simulink model "eval_ekf"  (R2026a)
settings: Solver=VariableStepAuto  StopTime=1000
undefined symbols (not defined in the file): ekf_param, pf_param, plant_param, r_param
libraries: lib_sensors x3, lib_plant x1
settings Model: SimulationMode=accelerator  Creator=alessandro-nardin  LastModifiedBy=alessandro-nardin
settings RTWCC: Toolchain=Microsoft Visual C++ 2022 v17.0 | nmake (64-bit Windows)

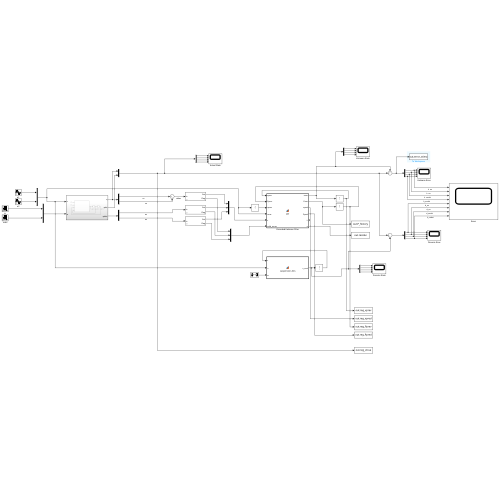
[thumbnail: Simulink's stored preview of the top-level diagram]
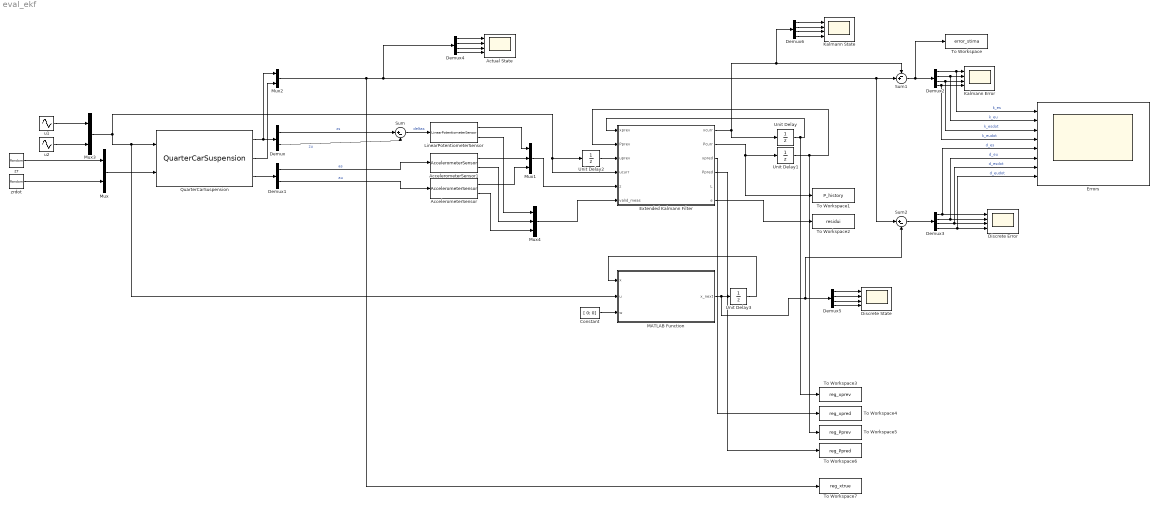
== system eval_ekf ==
  AccelerometerSensor : lib_sensors/AccelerometerSensor  out_sample_t=1/ekf_param.freq
  AccelerometerSensor1 : lib_sensors/AccelerometerSensor  out_sample_t=1/ekf_param.freq
  Actual State : Scope  NumInputPorts=4
      settings: ActiveDisplayYMinimum=-13.406936930450598  ActiveDisplayYMaximum=16.431517639223237  DataLoggingVariableName=ScopeData2
  Constant : Constant  Value=[ 0; 0]
  Demux : Demux  Outputs=2
  Demux1 : Demux  Outputs=2
  Demux{2..6} (5 alike) : Demux
  Discrete Error : Scope  NumInputPorts=4
      settings: ActiveDisplayYMinimum=-0.13461336894615539  ActiveDisplayYMaximum=0.12972172873522425
  Discrete State : Scope  NumInputPorts=4
      settings: ActiveDisplayYMinimum=-16.662431963356159  ActiveDisplayYMaximum=16.863664846001409  DataLoggingVariableName=ScopeData3
  Errors : Scope  NumInputPorts=8
      settings: ActiveDisplayYMinimum=-0.11152200034289453  ActiveDisplayYMaximum=0.13726275911567587  DataLoggingVariableName=ScopeData5
  Extended Kalmann Filter : MATLAB Function  TreatAsAtomicUnit=on
  Kalmann Error : Scope  NumInputPorts=4
      settings: ActiveDisplayYMinimum=-0.727367767410682  ActiveDisplayYMaximum=0.68734917974136311
  Kalmann State : Scope  NumInputPorts=4
      settings: ActiveDisplayYMinimum=-12.347879763067127  ActiveDisplayYMaximum=15.301795380492928  DataLoggingVariableName=ScopeData4
  LinearPotentiometerSensor : lib_sensors/LinearPotentiometerSensor  out_sample_t=1/ekf_param.freq
  MATLAB Function : MATLAB Function  TreatAsAtomicUnit=on
  Mux : Mux  Inputs=2
  Mux1 : Mux  Inputs=3
  Mux2 : Mux  Inputs=2
  Mux3 : Mux  Inputs=2
  Mux4 : Mux  Inputs=3
  QuarterCarSuspension : lib_plant/QuarterCarSuspension  SystemSampleTime=-1  VariantActivationTime=update diagram  EmptyChoice=off  PassThrough=off  PassThroughVariantControl=(default)  EmptyChoiceVariantControl=(default)  AllowFlexibleInterface=on  Latency=0  AutoFrameSizeCalculation=off
      settings: SourceProductName=Lib Plant
  Sum : Sum  Inputs=|+-
  Sum1 : Sum  Inputs=-+|
  Sum2 : Sum  Inputs=|+-
  To Workspace : ToWorkspace  VariableName=error_stima  SaveFormat=Timeseries  SampleTime=pf_param.sample_t
  To Workspace1 : ToWorkspace  VariableName=P_history  SaveFormat=Timeseries  SampleTime=-1
  To Workspace2 : ToWorkspace  VariableName=residui  SaveFormat=Timeseries  SampleTime=-1
  To Workspace3 : ToWorkspace  VariableName=reg_xprev  SaveFormat=Timeseries  SampleTime=1/ekf_param.freq
  To Workspace4 : ToWorkspace  VariableName=reg_xpred  SaveFormat=Timeseries  SampleTime=1/ekf_param.freq
  To Workspace5 : ToWorkspace  VariableName=reg_Pprev  SaveFormat=Timeseries  SampleTime=1/ekf_param.freq
  To Workspace6 : ToWorkspace  VariableName=reg_Ppred  SaveFormat=Timeseries  SampleTime=1/ekf_param.freq
  To Workspace7 : ToWorkspace  VariableName=reg_xtrue  SaveFormat=Timeseries  SampleTime=1/ekf_param.freq
  Unit Delay : UnitDelay  InitialCondition=ekf_param.x_init  SampleTime=ekf_param.sample_t
  Unit Delay1 : UnitDelay  InitialCondition=ekf_param.P_init  SampleTime=ekf_param.sample_t
  Unit Delay2 : UnitDelay  InitialCondition=[ 0; 0]  SampleTime=ekf_param.sample_t
  Unit Delay3 : UnitDelay  InitialCondition=ekf_param.x_init  SampleTime=-1
  u1 : Sin  Amplitude=943  Frequency=0.5  Phase=0.2  SampleTime=0
  u2 : Sin  Amplitude=2000  Phase=1  SampleTime=0
  zr : RandomNumber  Variance=r_param.rz_var  Seed=3245  SampleTime=0
  zrdot : RandomNumber  Variance=r_param.rzdot_var  Seed=213  SampleTime=0
  wires:
  QuarterCarSuspension/1 -> Demux/1, Mux2/1
  Demux/1 -> Sum/1  "zs"
  Demux/2 -> Sum/2  "zu"
  Sum/1 -> LinearPotentiometerSensor/1  "deltas"
  Demux1/2 -> AccelerometerSensor/1  "au"
  QuarterCarSuspension/3 -> Demux1/1
  Demux1/1 -> AccelerometerSensor1/1  "as"
  Mux/1 -> QuarterCarSuspension/2
  Extended Kalmann Filter/2(Pcurr) -> To Workspace1/1, Unit Delay1/1
  Unit Delay1/1 -> To Workspace5/1, Extended Kalmann Filter/2(Pprev)
  Mux3/1 -> QuarterCarSuspension/1, MATLAB Function/2(u), Extended Kalmann Filter/4(ucurr), Unit Delay2/1
  Unit Delay2/1 -> Extended Kalmann Filter/3(uprev)
  AccelerometerSensor1/1 -> Mux1/2
  Mux1/1 -> Extended Kalmann Filter/5(z)
  zr/1 -> Mux/1
  zrdot/1 -> Mux/2
  Unit Delay/1 -> To Workspace3/1, Extended Kalmann Filter/1(xprev)
  u1/1 -> Mux3/1
  u2/1 -> Mux3/2
  Unit Delay3/1 -> MATLAB Function/1(x)
  Constant/1 -> MATLAB Function/3(w)
  QuarterCarSuspension/2 -> Mux2/2
  Sum1/1 -> To Workspace/1, Demux2/1
  Demux2/1 -> Errors/1, Kalmann Error/1  "k_es"
  Demux2/2 -> Errors/2, Kalmann Error/2  "k_eu"
  Demux2/3 -> Errors/3, Kalmann Error/3  "k_esdot"
  Demux2/4 -> Errors/4, Kalmann Error/4  "k_eudot"
  Sum2/1 -> Demux3/1
  Demux3/4 -> Errors/8, Discrete Error/4  "d_eudot"
  Demux3/2 -> Errors/6, Discrete Error/2  "d_eu"
  Demux3/1 -> Errors/5, Discrete Error/1  "d_es"
  Demux3/3 -> Errors/7, Discrete Error/3  "d_esdot"
  Demux4/4 -> Actual State/4
  Mux2/1 -> To Workspace7/1, Demux4/1, Sum1/2, Sum2/1
  Demux4/2 -> Actual State/2
  Demux4/3 -> Actual State/3
  Demux4/1 -> Actual State/1
  Demux5/4 -> Discrete State/4
  MATLAB Function/1(x_next) -> Demux5/1, Sum2/2, Unit Delay3/1
  Demux5/2 -> Discrete State/2
  Demux5/3 -> Discrete State/3
  Demux5/1 -> Discrete State/1
  Demux6/4 -> Kalmann State/4
  Extended Kalmann Filter/1(xcurr) -> Unit Delay/1, Sum1/1, Demux6/1
  Demux6/2 -> Kalmann State/2
  Demux6/3 -> Kalmann State/3
  Demux6/1 -> Kalmann State/1
  AccelerometerSensor/1 -> Mux1/3
  Mux4/1 -> Extended Kalmann Filter/6(valid_meas)
  LinearPotentiometerSensor/2 -> Mux4/1
  AccelerometerSensor1/2 -> Mux4/2
  AccelerometerSensor/2 -> Mux4/3
  LinearPotentiometerSensor/1 -> Mux1/1
  Extended Kalmann Filter/6(e) -> To Workspace2/1
  Extended Kalmann Filter/3(xpred) -> To Workspace4/1
  Extended Kalmann Filter/4(Ppred) -> To Workspace6/1

== matlab function eval_ekf/MATLAB Function ==
  settings: updateMethod=DISCRETE  sampleTime=ekf_param.sample_t
  data: x input; u input; x_next output size=[ 4 1 ]; w input; plant_param parameter; ekf_param parameter
function x_next = suspension_dics( x, u, w, plant_param, ekf_param)
x_next = suspension_f_dics_euler( x, u, w, plant_param, ekf_param.sample_t);

== matlab function eval_ekf/Extended Kalmann Filter ==
  settings: updateMethod=DISCRETE  sampleTime=ekf_param.sample_t
  data: xprev input; Pprev input; uprev input; ucurr input; z input; xcurr output size=[ 4 1 ]; Pcurr output; xpred output; Ppred output; plant_param parameter; ekf_param parameter; L output; valid_meas input; e output
function [ xcurr, Pcurr, xpred, Ppred, L, e ] = ekf( xprev, Pprev, uprev, ucurr, z, plant_param, ekf_param, valid_meas)
[xcurr, Pcurr, xpred, Ppred, L,e] = ekf_step( xprev, Pprev, uprev, ucurr, z, plant_param, ekf_param, valid_meas);
